simulink model "user_io_board_controller_unconverted_backup"  (Simulink 6.3)
settings: Solver=ode45  StartTime=0.0  StopTime=20000  RelTol=1e-3
InitFcn:
  | init_lcd
StartFcn:
  | init_lcd
undefined symbols (not defined in the file): gcbh, xlBlockLoadCallback
libraries: xbsIndex_r4 x183
(part 1 of 3)
settings Model: LastModifiedBy=sgupta

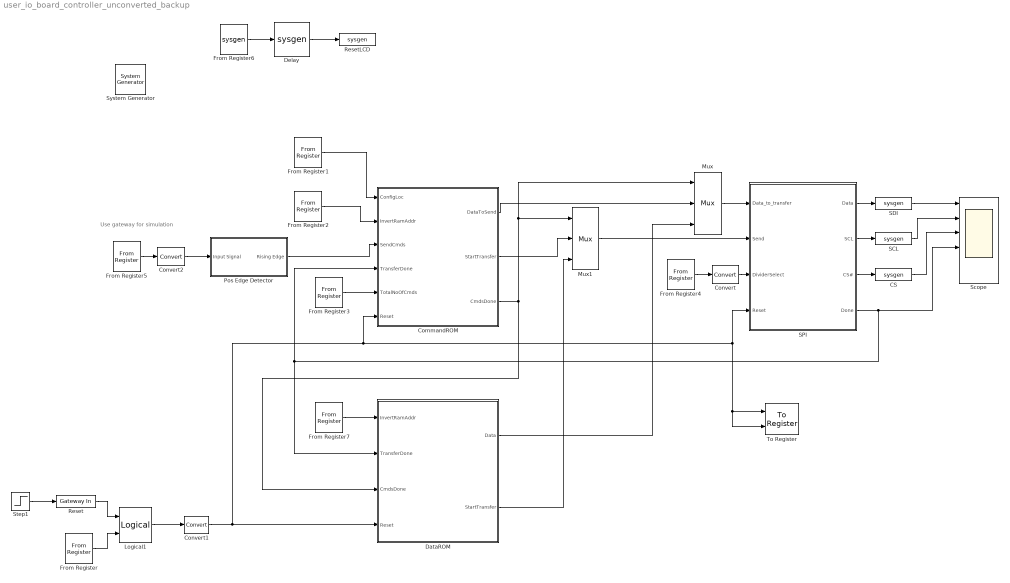
== system user_io_board_controller_unconverted_backup ==
  note: Use gateway for simulation
  " System Generator" : xbsIndex_r4/ System Generator  Tag=genX  xilinxfamily=Virtex4  part=xc4vsx35  speed=-10  package=ff668  synthesis_tool=XST  directory=./netlist  testbench=off  simulink_period=1  sysclk_period=10  incr_netlist=off  trim_vbits=Everywhere in SubSystem  dbl_ovrd=According to Block Masks  core_generation=According to Block Masks  run_coregen=off  deprecated_control=off  eval_field=0  block_type=sysgen
      settings: block_version=8.2.02
  CS : S-Function  LoadFcn=xlBlockLoadCallback(gcbh);  FunctionName=sysgen  Parameters=ptable_  mask(Xilinx Gateway Out Block){infoedit=Gateway out block.  Converts Xilinx fixed point inputs into ouputs of type Simulink integer, double, or fixed point.<P><P>Hardware notes:  In hardware these blocks become top level output ports or are discarded, depending on how they are configured., hdl_port_sgadvanced=, hdl_port=on, timing_constraint_sgadvanced=, timing_constraint=None, locs_specified_sgadvanced=, locs_specified=off, LOCs={}, xl_use_area_sgadvanced=, xl_use_area=off, xl_area=[0,0,0,0,0,0,0], sginterface=, has_advanced_control=0, sggui_pos=-1,-1,-1,-1, block_type=gatewayout, block_version=8.2.02, sg_icon_stat=60,20,1,1,white,yellow,0,f0cec300, sg_mask_display=|, sg_list_contents=, sg_blockgui_xml=|}
      mask sg_mask_display=|
      | fprintf('','COMMENT: begin icon graphics');
      | patch([0 60 60 0 ],[0 0 20 20 ],[0.95 0.93 0.65]);
      | patch([24 21 26 21 24 29 30 31 37 33 29 26 31 26 29 33 37 31 30 29 24 ],[2 5 10 15 18 18 17 18 18 14 18 15 10 5 2 6 2 2 3 2 2 ],[0.98 0.96 0.92]);
      | plot([0 0 60 60 0 ],[0 20 20 0 0 ]);
      | fprintf('','COMMENT: end icon graphics');
      | fprintf('','COMMENT: begin icon text');
      | color('black');port_label('input',1,' ');
      | color('black');port_label('output',1,'\fontsize{11pt}\bf Out ','texmode','on');
      | fprintf('','COMMENT: end icon text');
      mask sg_blockgui_xml=|
      | <!--   *  Copyright (c) 2005, Xilinx, Inc.  All Rights Reserved.           --><!--   *  Reproduction or reuse, in any form, without the explicit written --><!--   *  consent of Xilinx, Inc., is strictly prohibited.                 --><sysgenblock block_type="gatewayout" simulinkname="Gateway Out" >
      |  <icon width="60" bg_color="yellow" height="20" wmark_color="white" />
      |  <dll entry_point="gateway_out_config" name="Sysgen" />
      |  <handlers enablement="gatewayoutenablement" />
      |  <libraries>
      |   <library name="xbsIndex" />
      |   <library name="xbsBasic" />
      |   <library name="xbsTypes" />
      |  </libraries>
      |  <blockgui label="Xilinx Gateway Out" >
      |   <editbox evaluate="false" multi_line="true" name="infoedit" read_only="true" default="Gateway out block.  Converts Xilinx fixed point inputs into ouputs of type Simulink integer, double, or fixed point.&lt;P>&lt;P>Hardware notes:  In hardware these blocks become top level output ports or are discarded, depending on how they are configured." />
      |   <checkbox ctype="Int" evaluate="true" name="hdl_port" label="Translate into output port" default="on" />
      |   <radiogroup ctype="Int" evaluate="true" name="timing_constraint" label="IOB timing constraint" default="None" >
      |    <item value="None" label="None" />
      |    <item value="Data Rate" label="Data rate" />
      |    <item value="Data Rate;  Set 'FAST' Attribute" label="Data rate;  set 'FAST' attribute" />
      |   </radiogroup>
      |   <checkbox ctype="Int" evaluate="true" name="locs_specified" label="Specify IOB location constraints" default="off" />
      |   <editbox ctype="StringVector" evaluate="true" name="LOCs" label="IOB pad locations (cell array {'MSB', ..., 'LSB'})" default="{}" />
      |   <etch label="FPGA Area Estimation" >
      |    <checkbox name="xl_use_area" label="Define FPGA area for resource estimation" default="off" />
      |    <editbox top_label="true" name="xl_area" label="FPGA area [slices, FFs, BRAMs, LUTs, IOBs, emb. mults, TBUFs]" default="[0,0,0,0,0,0,0]" />
      |   </etch>
      |   <hiddenvar ctype="String" evaluate="false" name="sginterface" default="" />
      |  </blockgui>
      | </sysgenblock>
      mask prompts: infoedit ""; hdl_port_sgadvanced ""; hdl_port "Translate into output port"; timing_constraint_sgadvanced ""; timing_constraint "IOB timing constraint"; locs_specified_sgadvanced ""; locs_specified "Specify IOB location constraints"; LOCs "IOB pad locations (cell array {'MSB', ..., 'LSB'})"; xl_use_area_sgadvanced ""; xl_use_area "Define FPGA area for resource estimation"; xl_area "FPGA area [slices, FFs, BRAMs, LUTs, IOBs, emb. mults, TBUFs]"; sginterface ""; has_advanced_control ""; sggui_pos ""; block_type ""; block_version ""; sg_icon_stat ""; sg_mask_display ""; sg_list_contents ""; sg_blockgui_xml ""
      mask help:
      | Gateway out block.  Converts Xilinx fixed point inputs into ouputs of type Simulink integer, double, or fixed point.
      |
      | Hardware notes:  In hardware these blocks become top level output ports or are discarded, depending on how they are configured.
      mask init:
      | try
      |   tmp_gcb = gcb;
      |   tmp_gcbh = gcbh;
      |   xlMungeMaskParams;
      |   block_config = 'Sysgen:gateway_out_config';
      |   serialized_declarations = '{''LOCs''=>''StringVector'',''hdl_port''=>''Int'',''locs_specified''=>''Int'',''sginterface''=>''String'',''timing_constraint''=>''Int''}';
      |   ptable_ = xlblockprep(get_param(tmp_gcb, 'MaskWSVariables'));
      | catch
      |   global xl_report_errors;
      |   if(~isempty(xl_report_errors) && xl_report_errors)
      |     e = regexprep(lasterr, '\n', '\nError: ');
      |     disp(['Error: While running MaskInit code on block ' tmp_gcb ': ' e]);
      |     error(e);
      |   end
      | end
      settings: CopyFcn=xlBlockMoveCallback(gcbh);  DeleteFcn=xlDestroyGui(gcbh);  ModelCloseFcn=xlDestroyGui(gcbh);  PreSaveFcn=xlBlockPreSaveCallback(gcbh);  PostSaveFcn=xlBlockPostSaveCallback(gcbh);  DestroyFcn=xlDestroyGui(gcbh);  OpenFcn=xlOpenGui(gcbh, @gatewayoutenablement, -1)  CloseFcn=xlDestroyGui(gcbh);  MoveFcn=xlBlockMoveCallback(gcbh);
      mask Help: eval('xlWeb(xlhtmldoclink(''Gateway Out''))');
      mask StyleString: edit,edit,checkbox,edit,popup(None|Data Rate|Data Rate;  Set 'FAST' Attribute),edit,checkbox,edit,edit,checkbox,edit,edit,edit,edit,edit,edit,edit,edit,edit,edit
      mask Display:
      | fprintf('','COMMENT: begin icon graphics');
      | patch([0 60 60 0 ],[0 0 20 20 ],[0.95 0.93 0.65]);
      | patch([24 21 26 21 24 29 30 31 37 33 29 26 31 26 29 33 37 31 30 29 24 ],[2 5 10 15 18 18 17 18 18 14 18 15 10 5 2 6 2 2 3 2 2 ],[0.98 0.96 0.92]);
      | plot([0 0 60 60 0 ],[0 20 20 0 0 ]);
      | fprintf('','COMMENT: end icon graphics');
      | fprintf('','COMMENT: begin icon text');
      | color('black');port_label('input',1,' ');
      | color('black');port_label('output',1,'\fontsize{11pt}\bf Out ','texmode','on');
      | fprintf('','COMMENT: end icon text');
  CommandROM : Subsystem
  Convert : xbsIndex_r4/Convert  arith_type=Boolean  n_bits=16  bin_pt=14  quantization=Truncate  overflow=Wrap  latency=0  dbl_ovrd=off  pipeline=off  block_type=convert
      settings: block_version=8.2.02
  Convert1 : xbsIndex_r4/Convert  arith_type=Boolean  n_bits=16  bin_pt=14  quantization=Truncate  overflow=Wrap  latency=0  dbl_ovrd=off  pipeline=off  block_type=convert
      settings: block_version=8.2.02
  Convert2 : xbsIndex_r4/Convert  arith_type=Boolean  n_bits=16  bin_pt=14  quantization=Truncate  overflow=Wrap  latency=0  dbl_ovrd=off  pipeline=off  block_type=convert
      settings: block_version=8.2.02
  DataROM : Subsystem
  Delay : S-Function  LoadFcn=xlBlockLoadCallback(gcbh);  FunctionName=sysgen  Parameters=ptable_  mask(Xilinx Delay Block){infoedit=Hardware notes: A delay line is a chain, each link of which is an SRL16 followed by a flip-flop. If register retiming is enabled, the delay line is a chain of flip-flops., en_sgadvanced=, en=off, latency=4, dbl_ovrd_sgadvanced=, dbl_ovrd=off, reg_retiming_sgadvanced=, reg_retiming=off, xl_use_area_sgadvanced=, xl_use_area=off, xl_area=[0,0,0,0,0,0,0], has_advanced_control=0, sggui_pos=20,20,356,256, block_type=delay, block_version=8.2.02, sg_icon_stat=60,56,1,1,white,blue,0,c2217bc4, sg_mask_display=|, sg_list_contents=, sg_blockgui_xml=|}
      mask sg_mask_display=|
      | fprintf('','COMMENT: begin icon graphics');
      | patch([0 60 60 0 ],[0 0 56 56 ],[0.77 0.82 0.91]);
      | patch([15 6 19 6 15 30 34 38 54 41 29 20 32 20 29 41 54 38 34 30 15 ],[6 15 28 41 50 50 46 50 50 37 49 40 28 16 7 19 6 6 10 6 6 ],[0.98 0.96 0.92]);
      | plot([0 0 60 60 0 ],[0 56 56 0 0 ]);
      | fprintf('','COMMENT: end icon graphics');
      | fprintf('','COMMENT: begin icon text');
      | color('black');disp('z^{-4}','texmode','on');
      | fprintf('','COMMENT: end icon text');
      mask sg_blockgui_xml=|
      | <!--   *  Copyright (c) 2005, Xilinx, Inc.  All Rights Reserved.           --><!--   *  Reproduction or reuse, in any form, without the explicit written --><!--   *  consent of Xilinx, Inc., is strictly prohibited.                 --><sysgenblock block_type="delay" simulinkname="Delay" >
      |  <icon width="60" bg_color="blue" height="56" wmark_color="white" />
      |  <dll entry_point="Delay_config" name="Sysgen" />
      |  <handlers enablement="xlmagicenablement" />
      |  <libraries>
      |   <library name="xbsIndex" />
      |   <library name="xbsBasic" />
      |   <library name="xbsMemory" />
      |  </libraries>
      |  <blockgui label="Xilinx Delay" >
      |   <editbox evaluate="false" multi_line="true" name="infoedit" read_only="true" default="Hardware notes: A delay line is a chain, each link of which is an SRL16 followed by a flip-flop. If register retiming is enabled, the delay line is a chain of flip-flops." />
      |   <tabpane>
      |    <tab name="basictab" label="Basic" >
      |     <etch name="oportetch" label="Optional Ports" >
      |      <checkbox ctype="Int" evaluate="true" name="en" label="Provide enable port" default="off" />
      |     </etch>
      |     <editbox ctype="Int" evaluate="true" name="latency" label="Latency" default="1" />
      |    </tab>
      |    <tab name="advtab" label="Advanced" >
      |     <etch label="Simulation" >
      |      <checkbox ctype="Int" evaluate="true" name="dbl_ovrd" label="Override with doubles" default="off" />
      |     </etch>
      |    </tab>
      |    <tab name="impltab" label="Implementation" >
      |     <checkbox ctype="Int" evaluate="true" name="reg_retiming" label="Enable register retiming" default="off" />
      |     <etch label="FPGA Area Estimation" >
      |      <checkbox name="xl_use_area" label="Define FPGA area for resource estimation" default="off" />
      |      <editbox top_label="true" name="xl_area" label="FPGA area [slices, FFs, BRAMs, LUTs, IOBs, emb. mults, TBUFs]" default="[0,0,0,0,0,0,0]" />
      |     </etch>
      |    </tab>
      |   </tabpane>
      |  </blockgui>
      | </sysgenblock>
      mask prompts: infoedit ""; en_sgadvanced ""; en "Provide enable port"; dbl_ovrd_sgadvanced ""; dbl_ovrd "Override with doubles"; reg_retiming_sgadvanced ""; reg_retiming "Enable register retiming"; xl_use_area_sgadvanced ""; xl_use_area "Define FPGA area for resource estimation"; xl_area "FPGA area [slices, FFs, BRAMs, LUTs, IOBs, emb. mults, TBUFs]"; has_advanced_control ""; sggui_pos ""; block_type ""; block_version ""; sg_icon_stat ""; sg_mask_display ""; sg_list_contents ""; sg_blockgui_xml ""
      mask help: Hardware notes: A delay line is a chain, each link of which is an SRL16 followed by a flip-flop. If register retiming is enabled, the delay line is a chain of flip-flops.
      mask init:
      | try
      |   tmp_gcb = gcb;
      |   tmp_gcbh = gcbh;
      |   xlMungeMaskParams;
      |   block_config = 'Sysgen:Delay_config';
      |   serialized_declarations = '{''dbl_ovrd''=>''Int'',''en''=>''Int'',''latency''=>''Int'',''reg_retiming''=>''Int''}';
      |   ptable_ = xlblockprep(get_param(tmp_gcb, 'MaskWSVariables'));
      | catch
      |   global xl_report_errors;
      |   if(~isempty(xl_report_errors) && xl_report_errors)
      |     e = regexprep(lasterr, '\n', '\nError: ');
      |     disp(['Error: While running MaskInit code on block ' tmp_gcb ': ' e]);
      |     error(e);
      |   end
      | end
      settings: CopyFcn=xlBlockMoveCallback(gcbh);  DeleteFcn=xlDestroyGui(gcbh);  ModelCloseFcn=xlDestroyGui(gcbh);  PreSaveFcn=xlBlockPreSaveCallback(gcbh);  PostSaveFcn=xlBlockPostSaveCallback(gcbh);  DestroyFcn=xlDestroyGui(gcbh);  OpenFcn=xlOpenGui(gcbh, @xlmagicenablement, -1)  CloseFcn=xlDestroyGui(gcbh);  MoveFcn=xlBlockMoveCallback(gcbh);
      mask Help: eval('xlWeb(xlhtmldoclink(''Delay''))');
      mask Display:
      | fprintf('','COMMENT: begin icon graphics');
      | patch([0 60 60 0 ],[0 0 56 56 ],[0.77 0.82 0.91]);
      | patch([15 6 19 6 15 30 34 38 54 41 29 20 32 20 29 41 54 38 34 30 15 ],[6 15 28 41 50 50 46 50 50 37 49 40 28 16 7 19 6 6 10 6 6 ],[0.98 0.96 0.92]);
      | plot([0 0 60 60 0 ],[0 56 56 0 0 ]);
      | fprintf('','COMMENT: end icon graphics');
      | fprintf('','COMMENT: begin icon text');
      | color('black');disp('z^{-4}','texmode','on');
      | fprintf('','COMMENT: end icon text');
  From Register : xbsIndex_r4/From Register  shared_memory_name='LCD_Reset'  init=0  period=1  ownership=Locally owned and initialized  arith_type=Unsigned  n_bits=1  bin_pt=0  dbl_ovrd=off  block_type=fromreg
      settings: AttributesFormatString=From Register\n<< %<shared_memory_name> >>  infoedit="Register block that reads data to a shared memory register.  Delay of one sample period."  block_version=8.2.02
  From Register1 : xbsIndex_r4/From Register  shared_memory_name='LCD_ConfigLocation'  init=0  period=1  ownership=Locally owned and initialized  arith_type=Unsigned  n_bits=2  bin_pt=0  dbl_ovrd=off  block_type=fromreg
      settings: AttributesFormatString=From Register\n<< %<shared_memory_name> >>  infoedit="Register block that reads data to a shared memory register.  Delay of one sample period."  block_version=8.2.02
  From Register2 : xbsIndex_r4/From Register  shared_memory_name='LCD_InvertRAMAddrCmd'  init=0  period=1  ownership=Locally owned and initialized  arith_type=Unsigned  n_bits=1  bin_pt=0  dbl_ovrd=off  block_type=fromreg
      settings: AttributesFormatString=From Register\n<< %<shared_memory_name> >>  infoedit="Register block that reads data to a shared memory register.  Delay of one sample period."  block_version=8.2.02
  From Register3 : xbsIndex_r4/From Register  shared_memory_name='LCD_TotalCmdTransfer'  init=10  period=1  ownership=Locally owned and initialized  arith_type=Unsigned  n_bits=8  bin_pt=0  dbl_ovrd=off  block_type=fromreg
      settings: AttributesFormatString=From Register\n<< %<shared_memory_name> >>  infoedit="Register block that reads data to a shared memory register.  Delay of one sample period."  block_version=8.2.02
  From Register4 : xbsIndex_r4/From Register  shared_memory_name='LCD_DividerSelect'  init=0  period=1  ownership=Locally owned and initialized  arith_type=Unsigned  n_bits=1  bin_pt=0  dbl_ovrd=off  block_type=fromreg
      settings: AttributesFormatString=From Register\n<< %<shared_memory_name> >>  infoedit="Register block that reads data to a shared memory register.  Delay of one sample period."  block_version=8.2.02
  From Register5 : xbsIndex_r4/From Register  shared_memory_name='LCD_Send'  init=0  period=1  ownership=Locally owned and initialized  arith_type=Unsigned  n_bits=1  bin_pt=0  dbl_ovrd=off  block_type=fromreg
      settings: AttributesFormatString=From Register\n<< %<shared_memory_name> >>  infoedit="Register block that reads data to a shared memory register.  Delay of one sample period."  block_version=8.2.02
  From Register6 : S-Function  LoadFcn=xlBlockLoadCallback(gcbh);  FunctionName=sysgen  Parameters=ptable_  mask(Xilinx Shared Memory Based From Register Block){infoedit=Register block that reads data to a shared memory register.  Delay of one sample period., shared_memory_name='LCD_ResetLCD', init=1, period=1, ownership_sgadvanced=, ownership=Locally owned and initialized, arith_type_sgadvanced=, arith_type=Unsigned, n_bits=1, bin_pt=0, dbl_ovrd_sgadvanced=, dbl_ovrd=off, xl_use_area_sgadvanced=, xl_use_area=off, xl_area=[0,0,0,0,0,0,0], has_advanced_control=0, sggui_pos=20,20,379,246, block_type=fromreg, block_version=8.2.02, sg_icon_stat=45,50,0,1,white,blue,0,137b37a7, sg_mask_display=|, sg_list_contents=, sg_blockgui_xml=|}
      mask sg_mask_display=|
      | fprintf('','COMMENT: begin icon graphics');
      | patch([0 45 45 0 ],[0 0 50 50 ],[0.77 0.82 0.91]);
      | patch([10 3 14 3 10 22 25 28 41 31 21 14 25 14 21 31 41 28 25 22 10 ],[7 14 25 36 43 43 40 43 43 33 43 36 25 14 7 17 7 7 10 7 7 ],[0.98 0.96 0.92]);
      | plot([0 0 45 45 0 ],[0 50 50 0 0 ]);
      | fprintf('','COMMENT: end icon graphics');
      | fprintf('','COMMENT: begin icon text');
      | color('black');port_label('output',1,'dout');
      | fprintf('','COMMENT: end icon text');
      mask sg_blockgui_xml=|
      | <!--   *  Copyright (c) 2005, Xilinx, Inc.  All Rights Reserved.           --><!--   *  Reproduction or reuse, in any form, without the explicit written --><!--   *  consent of Xilinx, Inc., is strictly prohibited.                 --><sysgenblock block_type="fromreg" simulinkname="From Register" >
      |  <initialization file="xlfromreg_init.m" />
      |  <icon width="45" bg_color="blue" height="50" caption_format="From Register\n&lt;&lt; %&lt;shared_memory_name> >>" wmark_color="white" />
      |  <dll entry_point="fromreg_config" name="Sysgen" />
      |  <handlers enablement="fromregenablement" />
      |  <libraries>
      |   <library name="xbsIndex" />
      |   <library name="xbsShared" />
      |  </libraries>
      |  <blockgui label="Xilinx Shared Memory Based From Register" >
      |   <editbox evaluate="false" multi_line="true" name="infoedit" read_only="true" default="Register block that reads data to a shared memory register.  Delay of one sample period." />
      |   <tabpane>
      |    <tab name="basictab" label="Basic" >
      |     <editbox ctype="String" evaluate="true" name="shared_memory_name" label="Shared memory name" default="'Bar'" />
      |     <editbox ctype="Double" evaluate="true" name="init" label="Initial value" default="0" />
      |     <editbox ctype="Double" evaluate="true" name="period" label="Sample period" default="1" />
      |     <radiogroup ctype="Int" evaluate="true" name="ownership" label="Ownership and initialization" default="Owned and initialized elsewhere" >
      |      <item value="Locally owned and initialized" />
      |      <item value="Owned and initialized elsewhere" />
      |     </radiogroup>
      |    </tab>
      |    <tab name="typetab" label="Output Type" >
      |     <etch label="Output Precision" >
      |      <radiogroup ctype="Int" evaluate="true" name="arith_type" label="Output type" default="Signed  (2's comp)" >
      |       <item value="Signed  (2's comp)" label="Signed  (2's comp)" />
      |       <item value="Unsigned" label="Unsigned" />
      |      </radiogroup>
      |      <editbox ctype="Int" evaluate="true" name="n_bits" label="Number of bits" default="16" />
      |      <editbox ctype="Int" evaluate="true" name="bin_pt" label="Binary point" default="14" />
      |     </etch>
      |    </tab>
      |    <tab name="advtab" label="Advanced" >
      |     <etch label="Simulation" >
      |      <checkbox ctype="Int" evaluate="true" name="dbl_ovrd" label="Override with doubles" default="off" />
      |     </etch>
      |    </tab>
      |    <tab name="impltab" label="Implementation" >
      |     <etch label="FPGA Area Estimation" >
      |      <checkbox name="xl_use_area" label="Define FPGA area for resource estimation" default="off" />
      |      <editbox top_label="true" name="xl_area" label="FPGA area [slices, FFs, BRAMs, LUTs, IOBs, emb. mults, TBUFs]" default="[0,0,0,0,0,0,0]" />
      |     </etch>
      |    </tab>
      |   </tabpane>
      |  </blockgui>
      | </sysgenblock>
      mask prompts: infoedit ""; shared_memory_name "Shared memory name"; init "Initial value"; period "Sample period"; ownership_sgadvanced ""; ownership "Ownership and initialization"; arith_type_sgadvanced ""; arith_type "Output type"; n_bits "Number of bits"; bin_pt "Binary point"; dbl_ovrd_sgadvanced ""; dbl_ovrd "Override with doubles"; xl_use_area_sgadvanced ""; xl_use_area "Define FPGA area for resource estimation"; xl_area "FPGA area [slices, FFs, BRAMs, LUTs, IOBs, emb. mults, TBUFs]"; has_advanced_control ""; sggui_pos ""; block_type ""; block_version ""; sg_icon_stat ""; sg_mask_display ""; sg_list_contents ""; sg_blockgui_xml ""
      mask help: Register block that reads data to a shared memory register. Delay of one sample period.
      mask init:
      | try
      |   tmp_gcb = gcb;
      |   tmp_gcbh = gcbh;
      |   xlMungeMaskParams;
      |   block_config = 'Sysgen:fromreg_config';
      |   serialized_declarations = '{''arith_type''=>''Int'',''bin_pt''=>''Int'',''dbl_ovrd''=>''Int'',''init''=>''Double'',''n_bits''=>''Int'',''ownership''=>''Int'',''period''=>''Double'',''shared_memory_name''=>''String''}';
      |   xlfromreg_init();
      |   ptable_ = xlblockprep(get_param(tmp_gcb, 'MaskWSVariables'));
      | catch
      |   global xl_report_errors;
      |   if(~isempty(xl_report_errors) && xl_report_errors)
      |     e = regexprep(lasterr, '\n', '\nError: ');
      |     disp(['Error: While running MaskInit code on block ' tmp_gcb ': ' e]);
      |     error(e);
      |   end
      | end
      settings: AttributesFormatString=From Register\n<< %<shared_memory_name> >>  CopyFcn=xlBlockMoveCallback(gcbh);  DeleteFcn=xlDestroyGui(gcbh);  ModelCloseFcn=xlDestroyGui(gcbh);  PreSaveFcn=xlBlockPreSaveCallback(gcbh);  PostSaveFcn=xlBlockPostSaveCallback(gcbh);  DestroyFcn=xlDestroyGui(gcbh);  OpenFcn=xlOpenGui(gcbh, @fromregenablement, -1)  CloseFcn=xlDestroyGui(gcbh);  MoveFcn=xlBlockMoveCallback(gcbh);
      mask Help: eval('xlWeb(xlhtmldoclink(''From Register''))');
      mask StyleString: edit,edit,edit,edit,edit,popup(Locally owned and initialized|Owned and initialized elsewhere),edit,popup(Signed  (2's comp)|Unsigned),edit,edit,edit,checkbox,edit,checkbox,edit,edit,edit,edit,edit,edit,edit,edit,edit
      mask Display:
      | fprintf('','COMMENT: begin icon graphics');
      | patch([0 45 45 0 ],[0 0 50 50 ],[0.77 0.82 0.91]);
      | patch([10 3 14 3 10 22 25 28 41 31 21 14 25 14 21 31 41 28 25 22 10 ],[7 14 25 36 43 43 40 43 43 33 43 36 25 14 7 17 7 7 10 7 7 ],[0.98 0.96 0.92]);
      | plot([0 0 45 45 0 ],[0 50 50 0 0 ]);
      | fprintf('','COMMENT: end icon graphics');
      | fprintf('','COMMENT: begin icon text');
      | color('black');port_label('output',1,'dout');
      | fprintf('','COMMENT: end icon text');
  From Register7 : xbsIndex_r4/From Register  shared_memory_name='LCD_InvertRAMAddrData'  init=1  period=1  ownership=Locally owned and initialized  arith_type=Unsigned  n_bits=1  bin_pt=0  dbl_ovrd=off  block_type=fromreg
      settings: AttributesFormatString=From Register\n<< %<shared_memory_name> >>  infoedit="Register block that reads data to a shared memory register.  Delay of one sample period."  block_version=8.2.02
  Logical1 : xbsIndex_r4/Logical  logical_function=OR  inputs=2  en=off  latency=0  precision=Full  arith_type=Unsigned  n_bits=16  bin_pt=0  align_bp=on  dbl_ovrd=off  block_type=logical
      settings: block_version=8.2.02
  Mux : xbsIndex_r4/Mux  inputs=2  en=off  latency=0  precision=Full  arith_type=Unsigned  n_bits=16  bin_pt=14  quantization=Truncate  overflow=Wrap  dbl_ovrd=off  block_type=mux
      settings: block_version=8.2.02
  Mux1 : xbsIndex_r4/Mux  inputs=2  en=off  latency=0  precision=Full  arith_type=Unsigned  n_bits=16  bin_pt=14  quantization=Truncate  overflow=Wrap  dbl_ovrd=off  block_type=mux
      settings: block_version=8.2.02
  Pos Edge Detector : Subsystem
  Reset : xbsIndex_r4/Gateway In  arith_type=Unsigned  n_bits=1  bin_pt=0  quantization=Truncate  overflow=Wrap  period=1  dbl_ovrd=off  timing_constraint=None  locs_specified=off  LOCs={}  block_type=gatewayin
      settings: infoedit="Gateway in block.  Converts inputs of type Simulink integer, double and fixed point to  Xilinx fixed point type.<P><P>Hardware notes:  In hardware these blocks become top level input ports."  block_version=8.2.02
  ResetLCD : S-Function  LoadFcn=xlBlockLoadCallback(gcbh);  FunctionName=sysgen  Parameters=ptable_  mask(Xilinx Gateway Out Block){infoedit=Gateway out block.  Converts Xilinx fixed point inputs into ouputs of type Simulink integer, double, or fixed point.<P><P>Hardware notes:  In hardware these blocks become top level output ports or are discarded, depending on how they are configured., hdl_port_sgadvanced=, hdl_port=on, timing_constraint_sgadvanced=, timing_constraint=None, locs_specified_sgadvanced=, locs_specified=off, LOCs={}, xl_use_area_sgadvanced=, xl_use_area=off, xl_area=[0,0,0,0,0,0,0], sginterface=, has_advanced_control=0, sggui_pos=-1,-1,-1,-1, block_type=gatewayout, block_version=8.2.02, sg_icon_stat=60,20,1,1,white,yellow,0,f0cec300, sg_mask_display=|, sg_list_contents=, sg_blockgui_xml=|}
      mask sg_mask_display=|
      | fprintf('','COMMENT: begin icon graphics');
      | patch([0 60 60 0 ],[0 0 20 20 ],[0.95 0.93 0.65]);
      | patch([24 21 26 21 24 29 30 31 37 33 29 26 31 26 29 33 37 31 30 29 24 ],[2 5 10 15 18 18 17 18 18 14 18 15 10 5 2 6 2 2 3 2 2 ],[0.98 0.96 0.92]);
      | plot([0 0 60 60 0 ],[0 20 20 0 0 ]);
      | fprintf('','COMMENT: end icon graphics');
      | fprintf('','COMMENT: begin icon text');
      | color('black');port_label('input',1,' ');
      | color('black');port_label('output',1,'\fontsize{11pt}\bf Out ','texmode','on');
      | fprintf('','COMMENT: end icon text');
      mask sg_blockgui_xml=|
      | <!--   *  Copyright (c) 2005, Xilinx, Inc.  All Rights Reserved.           --><!--   *  Reproduction or reuse, in any form, without the explicit written --><!--   *  consent of Xilinx, Inc., is strictly prohibited.                 --><sysgenblock block_type="gatewayout" simulinkname="Gateway Out" >
      |  <icon width="60" bg_color="yellow" height="20" wmark_color="white" />
      |  <dll entry_point="gateway_out_config" name="Sysgen" />
      |  <handlers enablement="gatewayoutenablement" />
      |  <libraries>
      |   <library name="xbsIndex" />
      |   <library name="xbsBasic" />
      |   <library name="xbsTypes" />
      |  </libraries>
      |  <blockgui label="Xilinx Gateway Out" >
      |   <editbox evaluate="false" multi_line="true" name="infoedit" read_only="true" default="Gateway out block.  Converts Xilinx fixed point inputs into ouputs of type Simulink integer, double, or fixed point.&lt;P>&lt;P>Hardware notes:  In hardware these blocks become top level output ports or are discarded, depending on how they are configured." />
      |   <checkbox ctype="Int" evaluate="true" name="hdl_port" label="Translate into output port" default="on" />
      |   <radiogroup ctype="Int" evaluate="true" name="timing_constraint" label="IOB timing constraint" default="None" >
      |    <item value="None" label="None" />
      |    <item value="Data Rate" label="Data rate" />
      |    <item value="Data Rate;  Set 'FAST' Attribute" label="Data rate;  set 'FAST' attribute" />
      |   </radiogroup>
      |   <checkbox ctype="Int" evaluate="true" name="locs_specified" label="Specify IOB location constraints" default="off" />
      |   <editbox ctype="StringVector" evaluate="true" name="LOCs" label="IOB pad locations (cell array {'MSB', ..., 'LSB'})" default="{}" />
      |   <etch label="FPGA Area Estimation" >
      |    <checkbox name="xl_use_area" label="Define FPGA area for resource estimation" default="off" />
      |    <editbox top_label="true" name="xl_area" label="FPGA area [slices, FFs, BRAMs, LUTs, IOBs, emb. mults, TBUFs]" default="[0,0,0,0,0,0,0]" />
      |   </etch>
      |   <hiddenvar ctype="String" evaluate="false" name="sginterface" default="" />
      |  </blockgui>
      | </sysgenblock>
      mask prompts: infoedit ""; hdl_port_sgadvanced ""; hdl_port "Translate into output port"; timing_constraint_sgadvanced ""; timing_constraint "IOB timing constraint"; locs_specified_sgadvanced ""; locs_specified "Specify IOB location constraints"; LOCs "IOB pad locations (cell array {'MSB', ..., 'LSB'})"; xl_use_area_sgadvanced ""; xl_use_area "Define FPGA area for resource estimation"; xl_area "FPGA area [slices, FFs, BRAMs, LUTs, IOBs, emb. mults, TBUFs]"; sginterface ""; has_advanced_control ""; sggui_pos ""; block_type ""; block_version ""; sg_icon_stat ""; sg_mask_display ""; sg_list_contents ""; sg_blockgui_xml ""
      mask help:
      | Gateway out block.  Converts Xilinx fixed point inputs into ouputs of type Simulink integer, double, or fixed point.
      |
      | Hardware notes:  In hardware these blocks become top level output ports or are discarded, depending on how they are configured.
      mask init: same as user_io_board_controller_unconverted_backup/CS
      settings: CopyFcn=xlBlockMoveCallback(gcbh);  DeleteFcn=xlDestroyGui(gcbh);  ModelCloseFcn=xlDestroyGui(gcbh);  PreSaveFcn=xlBlockPreSaveCallback(gcbh);  PostSaveFcn=xlBlockPostSaveCallback(gcbh);  DestroyFcn=xlDestroyGui(gcbh);  OpenFcn=xlOpenGui(gcbh, @gatewayoutenablement, -1)  CloseFcn=xlDestroyGui(gcbh);  MoveFcn=xlBlockMoveCallback(gcbh);
      mask Help: eval('xlWeb(xlhtmldoclink(''Gateway Out''))');
      mask StyleString: edit,edit,checkbox,edit,popup(None|Data Rate|Data Rate;  Set 'FAST' Attribute),edit,checkbox,edit,edit,checkbox,edit,edit,edit,edit,edit,edit,edit,edit,edit,edit
      mask Display:
      | fprintf('','COMMENT: begin icon graphics');
      | patch([0 60 60 0 ],[0 0 20 20 ],[0.95 0.93 0.65]);
      | patch([24 21 26 21 24 29 30 31 37 33 29 26 31 26 29 33 37 31 30 29 24 ],[2 5 10 15 18 18 17 18 18 14 18 15 10 5 2 6 2 2 3 2 2 ],[0.98 0.96 0.92]);
      | plot([0 0 60 60 0 ],[0 20 20 0 0 ]);
      | fprintf('','COMMENT: end icon graphics');
      | fprintf('','COMMENT: begin icon text');
      | color('black');port_label('input',1,' ');
      | color('black');port_label('output',1,'\fontsize{11pt}\bf Out ','texmode','on');
      | fprintf('','COMMENT: end icon text');
  SCL : S-Function  LoadFcn=xlBlockLoadCallback(gcbh);  FunctionName=sysgen  Parameters=ptable_  mask(Xilinx Gateway Out Block){infoedit=Gateway out block.  Converts Xilinx fixed point inputs into ouputs of type Simulink integer, double, or fixed point.<P><P>Hardware notes:  In hardware these blocks become top level output ports or are discarded, depending on how they are configured., hdl_port_sgadvanced=, hdl_port=on, timing_constraint_sgadvanced=, timing_constraint=None, locs_specified_sgadvanced=, locs_specified=off, LOCs={}, xl_use_area_sgadvanced=, xl_use_area=off, xl_area=[0,0,0,0,0,0,0], sginterface=, has_advanced_control=0, sggui_pos=-1,-1,-1,-1, block_type=gatewayout, block_version=8.2.02, sg_icon_stat=60,20,1,1,white,yellow,0,f0cec300, sg_mask_display=|, sg_list_contents=, sg_blockgui_xml=|}
      mask sg_mask_display=|
      | fprintf('','COMMENT: begin icon graphics');
      | patch([0 60 60 0 ],[0 0 20 20 ],[0.95 0.93 0.65]);
      | patch([24 21 26 21 24 29 30 31 37 33 29 26 31 26 29 33 37 31 30 29 24 ],[2 5 10 15 18 18 17 18 18 14 18 15 10 5 2 6 2 2 3 2 2 ],[0.98 0.96 0.92]);
      | plot([0 0 60 60 0 ],[0 20 20 0 0 ]);
      | fprintf('','COMMENT: end icon graphics');
      | fprintf('','COMMENT: begin icon text');
      | color('black');port_label('input',1,' ');
      | color('black');port_label('output',1,'\fontsize{11pt}\bf Out ','texmode','on');
      | fprintf('','COMMENT: end icon text');
      mask sg_blockgui_xml=|
      | <!--   *  Copyright (c) 2005, Xilinx, Inc.  All Rights Reserved.           --><!--   *  Reproduction or reuse, in any form, without the explicit written --><!--   *  consent of Xilinx, Inc., is strictly prohibited.                 --><sysgenblock block_type="gatewayout" simulinkname="Gateway Out" >
      |  <icon width="60" bg_color="yellow" height="20" wmark_color="white" />
      |  <dll entry_point="gateway_out_config" name="Sysgen" />
      |  <handlers enablement="gatewayoutenablement" />
      |  <libraries>
      |   <library name="xbsIndex" />
      |   <library name="xbsBasic" />
      |   <library name="xbsTypes" />
      |  </libraries>
      |  <blockgui label="Xilinx Gateway Out" >
      |   <editbox evaluate="false" multi_line="true" name="infoedit" read_only="true" default="Gateway out block.  Converts Xilinx fixed point inputs into ouputs of type Simulink integer, double, or fixed point.&lt;P>&lt;P>Hardware notes:  In hardware these blocks become top level output ports or are discarded, depending on how they are configured." />
      |   <checkbox ctype="Int" evaluate="true" name="hdl_port" label="Translate into output port" default="on" />
      |   <radiogroup ctype="Int" evaluate="true" name="timing_constraint" label="IOB timing constraint" default="None" >
      |    <item value="None" label="None" />
      |    <item value="Data Rate" label="Data rate" />
      |    <item value="Data Rate;  Set 'FAST' Attribute" label="Data rate;  set 'FAST' attribute" />
      |   </radiogroup>
      |   <checkbox ctype="Int" evaluate="true" name="locs_specified" label="Specify IOB location constraints" default="off" />
      |   <editbox ctype="StringVector" evaluate="true" name="LOCs" label="IOB pad locations (cell array {'MSB', ..., 'LSB'})" default="{}" />
      |   <etch label="FPGA Area Estimation" >
      |    <checkbox name="xl_use_area" label="Define FPGA area for resource estimation" default="off" />
      |    <editbox top_label="true" name="xl_area" label="FPGA area [slices, FFs, BRAMs, LUTs, IOBs, emb. mults, TBUFs]" default="[0,0,0,0,0,0,0]" />
      |   </etch>
      |   <hiddenvar ctype="String" evaluate="false" name="sginterface" default="" />
      |  </blockgui>
      | </sysgenblock>
      mask prompts: infoedit ""; hdl_port_sgadvanced ""; hdl_port "Translate into output port"; timing_constraint_sgadvanced ""; timing_constraint "IOB timing constraint"; locs_specified_sgadvanced ""; locs_specified "Specify IOB location constraints"; LOCs "IOB pad locations (cell array {'MSB', ..., 'LSB'})"; xl_use_area_sgadvanced ""; xl_use_area "Define FPGA area for resource estimation"; xl_area "FPGA area [slices, FFs, BRAMs, LUTs, IOBs, emb. mults, TBUFs]"; sginterface ""; has_advanced_control ""; sggui_pos ""; block_type ""; block_version ""; sg_icon_stat ""; sg_mask_display ""; sg_list_contents ""; sg_blockgui_xml ""
      mask help:
      | Gateway out block.  Converts Xilinx fixed point inputs into ouputs of type Simulink integer, double, or fixed point.
      |
      | Hardware notes:  In hardware these blocks become top level output ports or are discarded, depending on how they are configured.
      mask init: same as user_io_board_controller_unconverted_backup/CS
      settings: CopyFcn=xlBlockMoveCallback(gcbh);  DeleteFcn=xlDestroyGui(gcbh);  ModelCloseFcn=xlDestroyGui(gcbh);  PreSaveFcn=xlBlockPreSaveCallback(gcbh);  PostSaveFcn=xlBlockPostSaveCallback(gcbh);  DestroyFcn=xlDestroyGui(gcbh);  OpenFcn=xlOpenGui(gcbh, @gatewayoutenablement, -1)  CloseFcn=xlDestroyGui(gcbh);  MoveFcn=xlBlockMoveCallback(gcbh);
      mask Help: eval('xlWeb(xlhtmldoclink(''Gateway Out''))');
      mask StyleString: edit,edit,checkbox,edit,popup(None|Data Rate|Data Rate;  Set 'FAST' Attribute),edit,checkbox,edit,edit,checkbox,edit,edit,edit,edit,edit,edit,edit,edit,edit,edit
      mask Display:
      | fprintf('','COMMENT: begin icon graphics');
      | patch([0 60 60 0 ],[0 0 20 20 ],[0.95 0.93 0.65]);
      | patch([24 21 26 21 24 29 30 31 37 33 29 26 31 26 29 33 37 31 30 29 24 ],[2 5 10 15 18 18 17 18 18 14 18 15 10 5 2 6 2 2 3 2 2 ],[0.98 0.96 0.92]);
      | plot([0 0 60 60 0 ],[0 20 20 0 0 ]);
      | fprintf('','COMMENT: end icon graphics');
      | fprintf('','COMMENT: begin icon text');
      | color('black');port_label('input',1,' ');
      | color('black');port_label('output',1,'\fontsize{11pt}\bf Out ','texmode','on');
      | fprintf('','COMMENT: end icon text');
  SDI : S-Function  LoadFcn=xlBlockLoadCallback(gcbh);  FunctionName=sysgen  Parameters=ptable_  mask(Xilinx Gateway Out Block){infoedit=Gateway out block.  Converts Xilinx fixed point inputs into ouputs of type Simulink integer, double, or fixed point.<P><P>Hardware notes:  In hardware these blocks become top level output ports or are discarded, depending on how they are configured., hdl_port_sgadvanced=, hdl_port=on, timing_constraint_sgadvanced=, timing_constraint=None, locs_specified_sgadvanced=, locs_specified=off, LOCs={}, xl_use_area_sgadvanced=, xl_use_area=off, xl_area=[0,0,0,0,0,0,0], sginterface=, has_advanced_control=0, sggui_pos=20,20,356,335, block_type=gatewayout, block_version=8.2.02, sg_icon_stat=60,20,1,1,white,yellow,0,f0cec300, sg_mask_display=|, sg_list_contents=, sg_blockgui_xml=|}
      mask sg_mask_display=|
      | fprintf('','COMMENT: begin icon graphics');
      | patch([0 60 60 0 ],[0 0 20 20 ],[0.95 0.93 0.65]);
      | patch([24 21 26 21 24 29 30 31 37 33 29 26 31 26 29 33 37 31 30 29 24 ],[2 5 10 15 18 18 17 18 18 14 18 15 10 5 2 6 2 2 3 2 2 ],[0.98 0.96 0.92]);
      | plot([0 0 60 60 0 ],[0 20 20 0 0 ]);
      | fprintf('','COMMENT: end icon graphics');
      | fprintf('','COMMENT: begin icon text');
      | color('black');port_label('input',1,' ');
      | color('black');port_label('output',1,'\fontsize{11pt}\bf Out ','texmode','on');
      | fprintf('','COMMENT: end icon text');
      mask sg_blockgui_xml=|
      | <!--   *  Copyright (c) 2005, Xilinx, Inc.  All Rights Reserved.           --><!--   *  Reproduction or reuse, in any form, without the explicit written --><!--   *  consent of Xilinx, Inc., is strictly prohibited.                 --><sysgenblock block_type="gatewayout" simulinkname="Gateway Out" >
      |  <icon width="60" bg_color="yellow" height="20" wmark_color="white" />
      |  <dll entry_point="gateway_out_config" name="Sysgen" />
      |  <handlers enablement="gatewayoutenablement" />
      |  <libraries>
      |   <library name="xbsIndex" />
      |   <library name="xbsBasic" />
      |   <library name="xbsTypes" />
      |  </libraries>
      |  <blockgui label="Xilinx Gateway Out" >
      |   <editbox evaluate="false" multi_line="true" name="infoedit" read_only="true" default="Gateway out block.  Converts Xilinx fixed point inputs into ouputs of type Simulink integer, double, or fixed point.&lt;P>&lt;P>Hardware notes:  In hardware these blocks become top level output ports or are discarded, depending on how they are configured." />
      |   <checkbox ctype="Int" evaluate="true" name="hdl_port" label="Translate into output port" default="on" />
      |   <radiogroup ctype="Int" evaluate="true" name="timing_constraint" label="IOB timing constraint" default="None" >
      |    <item value="None" label="None" />
      |    <item value="Data Rate" label="Data rate" />
      |    <item value="Data Rate;  Set 'FAST' Attribute" label="Data rate;  set 'FAST' attribute" />
      |   </radiogroup>
      |   <checkbox ctype="Int" evaluate="true" name="locs_specified" label="Specify IOB location constraints" default="off" />
      |   <editbox ctype="StringVector" evaluate="true" name="LOCs" label="IOB pad locations (cell array {'MSB', ..., 'LSB'})" default="{}" />
      |   <etch label="FPGA Area Estimation" >
      |    <checkbox name="xl_use_area" label="Define FPGA area for resource estimation" default="off" />
      |    <editbox top_label="true" name="xl_area" label="FPGA area [slices, FFs, BRAMs, LUTs, IOBs, emb. mults, TBUFs]" default="[0,0,0,0,0,0,0]" />
      |   </etch>
      |   <hiddenvar ctype="String" evaluate="false" name="sginterface" default="" />
      |  </blockgui>
      | </sysgenblock>
      mask prompts: infoedit ""; hdl_port_sgadvanced ""; hdl_port "Translate into output port"; timing_constraint_sgadvanced ""; timing_constraint "IOB timing constraint"; locs_specified_sgadvanced ""; locs_specified "Specify IOB location constraints"; LOCs "IOB pad locations (cell array {'MSB', ..., 'LSB'})"; xl_use_area_sgadvanced ""; xl_use_area "Define FPGA area for resource estimation"; xl_area "FPGA area [slices, FFs, BRAMs, LUTs, IOBs, emb. mults, TBUFs]"; sginterface ""; has_advanced_control ""; sggui_pos ""; block_type ""; block_version ""; sg_icon_stat ""; sg_mask_display ""; sg_list_contents ""; sg_blockgui_xml ""
      mask help:
      | Gateway out block.  Converts Xilinx fixed point inputs into ouputs of type Simulink integer, double, or fixed point.
      |
      | Hardware notes:  In hardware these blocks become top level output ports or are discarded, depending on how they are configured.
      mask init: same as user_io_board_controller_unconverted_backup/CS
      settings: CopyFcn=xlBlockMoveCallback(gcbh);  DeleteFcn=xlDestroyGui(gcbh);  ModelCloseFcn=xlDestroyGui(gcbh);  PreSaveFcn=xlBlockPreSaveCallback(gcbh);  PostSaveFcn=xlBlockPostSaveCallback(gcbh);  DestroyFcn=xlDestroyGui(gcbh);  OpenFcn=xlOpenGui(gcbh, @gatewayoutenablement, -1)  CloseFcn=xlDestroyGui(gcbh);  MoveFcn=xlBlockMoveCallback(gcbh);
      mask Help: eval('xlWeb(xlhtmldoclink(''Gateway Out''))');
      mask StyleString: edit,edit,checkbox,edit,popup(None|Data Rate|Data Rate;  Set 'FAST' Attribute),edit,checkbox,edit,edit,checkbox,edit,edit,edit,edit,edit,edit,edit,edit,edit,edit
      mask Display:
      | fprintf('','COMMENT: begin icon graphics');
      | patch([0 60 60 0 ],[0 0 20 20 ],[0.95 0.93 0.65]);
      | patch([24 21 26 21 24 29 30 31 37 33 29 26 31 26 29 33 37 31 30 29 24 ],[2 5 10 15 18 18 17 18 18 14 18 15 10 5 2 6 2 2 3 2 2 ],[0.98 0.96 0.92]);
      | plot([0 0 60 60 0 ],[0 20 20 0 0 ]);
      | fprintf('','COMMENT: end icon graphics');
      | fprintf('','COMMENT: begin icon text');
      | color('black');port_label('input',1,' ');
      | color('black');port_label('output',1,'\fontsize{11pt}\bf Out ','texmode','on');
      | fprintf('','COMMENT: end icon text');
  SPI : Subsystem
  Scope : Scope  NumInputPorts=6
      settings: YMin=-5~-5~-5~-5~-5~-5  YMax=5~5~5~5~5~5
  Step1 : Step  Time=10  Before=1  After=0  SampleTime=1
  To Register : xbsIndex_r4/To Register  shared_memory_name='LCD_Bar'  init=0  ownership=Locally owned and initialized  explicit_data_type=off  arith_type="Signed  (2's comp)"  n_bits=16  bin_pt=14  dbl_ovrd=off  block_type=toreg
      settings: AttributesFormatString=To Register\n<< %<shared_memory_name> >>  infoedit="Register block that writes data to a shared memory register.  Delay of one sample period."  block_version=8.2.02
  wires:
  Convert2/1 -> Pos Edge Detector/1(Input Signal)
  From Register1/1 -> CommandROM/1(ConfigLoc)
  From Register2/1 -> CommandROM/2(InvertRamAddr)
  Pos Edge Detector/1(Rising Edge) -> CommandROM/3(SendCmds)
  Convert/1 -> SPI/3(DividerSelect)
  SPI/4(Done) -> Scope/4, CommandROM/4(TransferDone), DataROM/2(TransferDone)
  SPI/1(Data) -> SDI/1
  SPI/2(SCL) -> SCL/1
  SPI/3(CS#) -> CS/1
  Step1/1 -> Reset/1
  Reset/1 -> Logical1/1
  From Register/1 -> Logical1/2
  Logical1/1 -> Convert1/1
  From Register3/1 -> CommandROM/5(TotalNoOfCmds)
  From Register4/1 -> Convert/1
  From Register6/1 -> Delay/1
  Delay/1 -> ResetLCD/1
  SDI/1 -> Scope/1
  SCL/1 -> Scope/2
  CS/1 -> Scope/3
  From Register7/1 -> DataROM/1(InvertRamAddr)
  CommandROM/3(CmdsDone) -> DataROM/3(CmdsDone), Mux1/1, Mux/1
  Convert1/1 -> DataROM/4(Reset), CommandROM/6(Reset), SPI/4(Reset), To Register/1, To Register/2
  Mux/1 -> SPI/1(Data_to_transfer)
  Mux1/1 -> SPI/2(Send)
  CommandROM/1(DataToSend) -> Mux/2
  CommandROM/2(StartTransfer) -> Mux1/2
  DataROM/1(Data) -> Mux/3
  DataROM/2(StartTransfer) -> Mux1/3
  From Register5/1 -> Convert2/1
